simulink model "H24_logicalSOC"  (R2023b)
settings: Solver=FixedStepAuto  StartTime=0.0  StopTime=TimeEnd  FixedStep=dTime  RelTol=1e-3
undefined symbols (not defined in the file): CoolInTemp
libraries: ESE_Saft_SL2A x1, BatteryLibrary_lib_YL x1
settings Model: Creator=Yi.Li  LastModifiedBy=Yi.Li

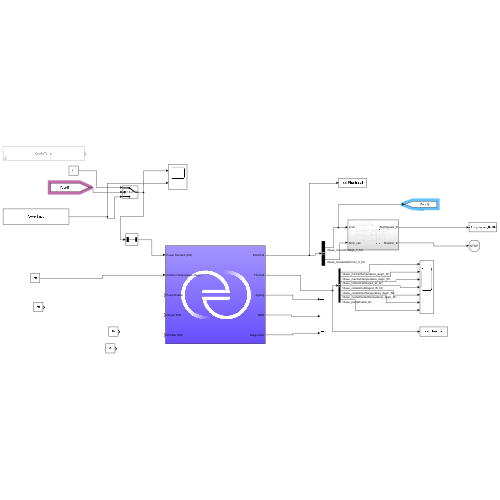
[thumbnail: Simulink's stored preview of the top-level diagram]
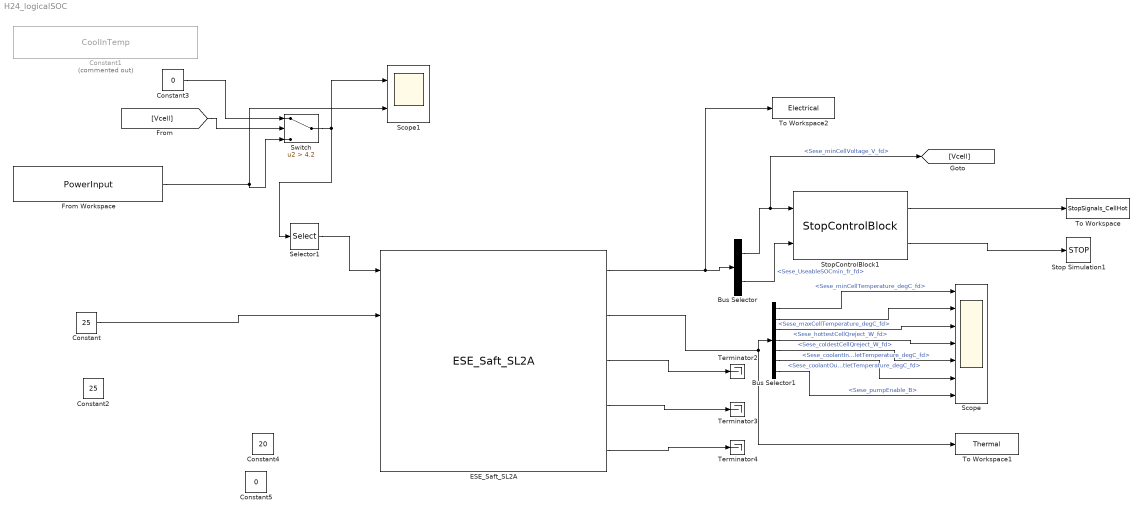
== system H24_logicalSOC ==
  Bus Selector : BusSelector  OutputSignals=Sese_minCellVoltage_V_fd,Sese_UseableSOCmin_fr_fd
  Bus Selector1 : BusSelector  OutputSignals=Sese_minCellTemperature_degC_fd,Sese_maxCellTemperature_degC_fd,Sese_hottestCellQreject_W_fd,Sese_coldestCellQreject_W_fd,Sese_coolantInletTemperature_degC_fd,Sese_coolantOutletTemperature_degC_fd,Sese_pumpEnable_B
  Constant : Constant  Value=25
  Constant1 : Constant  Commented=on  Value=CoolInTemp
  Constant2 : Constant  Value=25
  Constant3 : Constant  Value=0
  Constant4 : Constant  Value=20
  Constant5 : Constant  Value=0
  ESE_Saft_SL2A : ESE_Saft_SL2A/ESE_Saft_SL2A  modelSelect=Pack Concept  inputSelect=Power  thermalSelect=Outlet Estimated Model  electricalSelect=Full Cell ECN  ageingSelect=Semi-empirical Rainflow  applyPowerLimits=off  Pese_BalancingEnabled_B=on  Pese_BalancingCurrent_A_fd=0.05  Pese_cellTemperatureInit_degC_fd=CellPar.InitialCon.TempCellStart  Pese_SOCimbalance_fr_fd=CellPar.InitialCon.SOCImbalance  Pese_Thermalimbalance_degC_fd=CellPar.InitialCon.TempCellImbalance  Pese_SOCinit_fr_fd=SOCstart  Pese_Rweld_Ohm_fd=0  Pese_numSeries_Z_fd=Ns  Pese_numParallel_Z_fd=Np  Pese_LLI_pc_fd=0  Pese_LAM_an_pc_fd=0  Pese_LAM_ca_pc_fd=0  Pese_coolantFlowRate_lpm_fd=20  Pese_CpCoolant_Z_fd=CellPar.ThermalProperties.CoolCp  Pese_rhoCoolant_Z_fd=CellPar.ThermalProperties.CoolDensity  Pese_RthermalCelltoEnvironment_K_W_fd=CellPar.ThermalProperties.ThermalRes_CellEnv  Pese_RthermalCelltoCoolant_K_W_fd=InputPar.ThermalRes_CellCool  Pese_timehorizonsVec_s_fd="[1  2  5]"  Pese_USOCHi_fr_fd=0.97  Pese_USOCLo_fr_fd=0.02  Pese_UpperCellVoltageLimit_V_fd=4.25  Pese_LowerCellVoltageLimit_V_fd=2.7  Pese_AnodeVoltageLimit_V_fd=0.05  Pese_ILimMaxRegenVec_A_fd="[250  250  240]"  Pese_ILimMaxDchgVec_A_fd=[-360 -360 -360]  Pese_ILimMaxChgSocDerateLUTMtrx_fr_fd="[0.02         0.1         0.2         0.3         0.4        0.95           1;1  1  1  1  1  1  0]"  Pese_ILimMaxDchgSocDerateLUTMtrx_fr_fd="[0        0.08         0.1         0.2         0.3         0.4           1;0        0.25           1           1           1           1           1]"  Pese_ILimMaxTempDerateLUTMtrx_fr_fd="[-20   0  10  30  45  50  80  85  90;0           0           0         0.1         0.5           1           1           0           0]"  Pese_BMSdecimation_s_fd=1  Pese_SOH_Capacity_Init_Z_fd=1  Pese_DoDmin_pr_fd=2  Pese_ageingUpdateTime_s_fd=10  resGain=1  capGain=1  SOHc_StopCondition=0.8
  From Workspace : FromWorkspace  VariableName=PowerInput  SampleTime=-1  OutputAfterFinalValue=Holding final value
  Scope : Scope  NumInputPorts=7
  Scope1 : Scope  NumInputPorts=2
  Selector1 : Selector  InputPortWidth=1  IndexOptions=Index vector (dialog)  Indices=1  OutputSizes=1
  Stop Simulation1 : Stop
  StopControlBlock1 : BatteryLibrary_lib_YL/StopControlBlock  SystemSampleTime=-1  VariantActivationTime=update diagram  AllowFlexibleInterface=on  Latency=0  AutoFrameSizeCalculation=off
  Switch : Switch  Criteria=u2 > Threshold  Threshold=4.2  SaturateOnIntegerOverflow=off  InputSameDT=off
  Terminator2 : Terminator
  Terminator3 : Terminator
  Terminator4 : Terminator
  To Workspace : ToWorkspace  VariableName=StopSignals_CellHot  SaveFormat=Timeseries  SampleTime=-1
  To Workspace1 : ToWorkspace  VariableName=Thermal  SaveFormat=Timeseries  SampleTime=-1
  To Workspace2 : ToWorkspace  VariableName=Electrical  SaveFormat=Timeseries  SampleTime=-1
  wires:
  StopControlBlock1/2 -> Stop Simulation1/1
  ESE_Saft_SL2A/1 -> To Workspace2/1, Bus Selector/1
  Bus Selector/1 -> [Vcell], StopControlBlock1/1  "<Sese_minCellVoltage_V_fd>"
  StopControlBlock1/1 -> To Workspace/1
  Bus Selector/2 -> StopControlBlock1/2  "<Sese_UseableSOCmin_fr_fd>"
  ESE_Saft_SL2A/2 -> To Workspace1/1, Bus Selector1/1
  ESE_Saft_SL2A/3 -> Terminator2/1
  ESE_Saft_SL2A/4 -> Terminator3/1
  ESE_Saft_SL2A/5 -> Terminator4/1
  Bus Selector1/1 -> Scope/1  "<Sese_minCellTemperature_degC_fd>"
  Bus Selector1/2 -> Scope/2  "<Sese_maxCellTemperature_degC_fd>"
  Bus Selector1/3 -> Scope/3  "<Sese_hottestCellQreject_W_fd>"
  Bus Selector1/4 -> Scope/4  "<Sese_coldestCellQreject_W_fd>"
  Bus Selector1/5 -> Scope/5  "<Sese_coolantInletTemperature_degC_fd>"
  Bus Selector1/6 -> Scope/6  "<Sese_coolantOutletTemperature_degC_fd>"
  Bus Selector1/7 -> Scope/7  "<Sese_pumpEnable_B>"
  Constant/1 -> ESE_Saft_SL2A/2
  [Vcell] -> Switch/2
  Constant3/1 -> Switch/1
  From Workspace/1 -> Switch/3, Scope1/2
  Switch/1 -> Scope1/1, Selector1/1
  Selector1/1 -> ESE_Saft_SL2A/1
